simulink model "FTCSimulation_2023a"  (R2023a)
settings: Solver=FixedStepAuto  StartTime=0.0  StopTime=SimTime  FixedStep=0.01  RelTol=1e-3
values from neighbouring files (symbols this model uses):
  g = 9.81    [aero_guid_dat.m]
  Iyy = 182.5/(Kg2slug*m2ft^2)    (= 247.436636441)    [aero_guid_dat.m]
  L = 0.0065    [aero_guid_dat.m]
undefined symbols (not defined in the file or in its folder): A_x, A_y, A_z, AF, apSampleTime, arSampleTime, B_x, B_y, B_z, c_1, c_2, c_3, c_4, C_x, C_y, C_z, CAM, Continuous, D_x, D_y, D_z, Dis, ESO, GOSELM, inertia, Ixx, Izz, K_a1, K_a2, K_a3, K_d, K_d_LQR_phi, K_d_LQR_psi, K_d_LQR_theta, K_d_LQR_x, K_d_LQR_y, K_d_LQR_z, K_p1, K_p2, K_p3, K_q_LQR_phi, K_q_LQR_psi, K_q_LQR_theta, K_q_LQR_x, K_q_LQR_y, K_q_LQR_z, lambda, m, M, Noise, SM, Time
libraries: simulink x6, ctrlSharedLib x3, eeGeneralControl x1
(part 1 of 2)
settings Model: PacingRate=1.400000  Creator=Mahdi  LastModifiedBy=Mahdi
settings OptimizationCC: UseDivisionForNetSlopeComputation=on  GainParamInheritBuiltInType=on  UseFloatMulNetSlope=on  EnhancedBackFolding=on  PassReuseOutputArgsThreshold=0  MaxStackSize=64  OptimizeBlockOrder=speed  DifferentSizesBufferReuse=on  OptimizationCustomize=off
settings DebuggingCC: MultiTaskRateTransMsg=warning  ParameterTunabilityLossMsg=error  UnconnectedInputMsg=warning  UnconnectedOutputMsg=warning  UnconnectedLineMsg=warning
settings ModelReferenceCC: EnableRefExpFcnMdlSchedulingChecks=on
settings SFSimCC: MATLABDynamicMemAlloc=off
settings RTWCC: GenerateReport=on  BuildConfiguration=Faster Runs  LaunchReport=on  DLArmComputeVersion=19.05
settings CodeAppCC: ForceParamTrailComments=on  OperatorAnnotations=on  StateflowObjectComments=on
settings GRTTargetCC: TargetLangStandard=C89/C90 (ANSI)

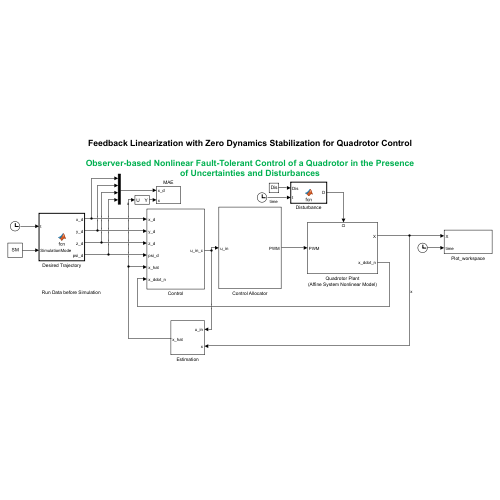
[thumbnail: Simulink's stored preview of the top-level diagram]
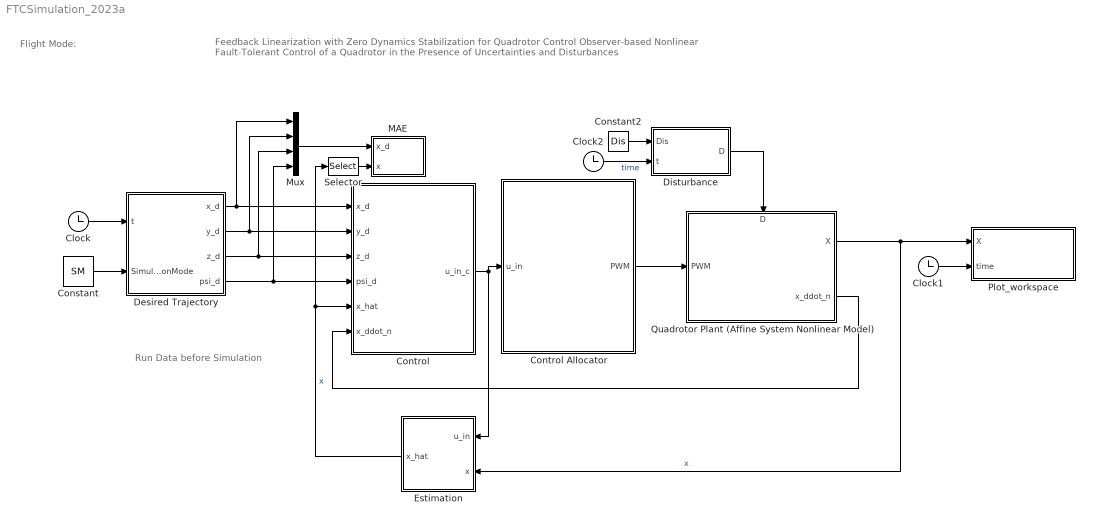
== system FTCSimulation_2023a ==
  note: Run Data before Simulation
  note: Flight Mode:
  note: Feedback Linearization with Zero Dynamics Stabilization for Quadrotor Control
      |
      | Observer-based Nonlinear Fault-Tolerant Control of a Quadrotor in the Presence of Uncertainties and Disturbances
  Clock : Clock
  Clock1 : Clock
  Clock2 : Clock
  Constant : Constant  Value=SM
  Constant2 : Constant  Value=Dis
  Control : Subsystem
  Control Allocator : Subsystem  SystemSampleTime=arSampleTime
  Desired Trajectory : MATLAB Function  TreatAsAtomicUnit=on
  Disturbance : MATLAB Function  TreatAsAtomicUnit=on
  Estimation : Subsystem  VariantControl=true
  MAE : Subsystem
  Mux : Mux
  Plot_workspace : Subsystem
  Quadrotor Plant (Affine System Nonlinear Model) : Subsystem  VariantControl=Choice_1
      settings: PortSchema="{\"entries\":[{\"content\":{\"sides\":[{\"content\":{\"connectorIds\":[\"In1\"]},\"type\":\"ConnectorPlacement.EquallySpacedRectSide\",\"uuid\":\"56cf6a8b-cd11-499a-8a7a-bce78fe94a21\"},{\"content\":{\"connectorIds\":[\"Out1\",\"Out2\"],\"side\":\"RIGHT\"},\"type\":\"ConnectorPlacement.EquallySpacedRectSide\",\"uuid\":\"b8074e7e-b572-4105-951c-798bb82723f6\"},{\"content\":{\"connectorIds\":[\"In2\"],\"side\":\"TOP\"},\"type\":\"ConnectorPlacement.EquallySpacedRectSide\",\"uuid\":\"331d9772-f954-417a-8685-e6b6106d3a97\"}]},\"type\":\"ConnectorPlacement.EquallySpacedConnector\",\"uuid\":\"13cb1b10-b6e3-4763-ba11-23de6fd316ae\"}],\"packageUris\":[\"http://schema.mathworks.com/mf0/Connector/R2020b\"],\"version\":\"1.0\"}"
  Selector : Selector  InputPortWidth=12  IndexOptions=Index vector (dialog)  Indices=[1 2 3 6]  OutputSizes=1
  wires:
  Control/1(u_in_c) -> Estimation/1(u_in), Control Allocator/1(u_in)
  Desired Trajectory/4(psi_d) -> Mux/4, Control/4(psi_d)
  Desired Trajectory/3(z_d) -> Mux/3, Control/3(z_d)
  Desired Trajectory/2(y_d) -> Mux/2, Control/2(y_d)
  Desired Trajectory/1(x_d) -> Mux/1, Control/1(x_d)
  Control Allocator/1(PWM) -> Quadrotor Plant (Affine System Nonlinear Model)/1(PWM)
  Quadrotor Plant (Affine System Nonlinear Model)/1(X) -> Estimation/2(x), Plot_workspace/1(X)  "x"
  Clock/1 -> Desired Trajectory/1(t)
  Constant/1 -> Desired Trajectory/2(SimulationMode)
  Clock1/1 -> Plot_workspace/2(time)
  Clock2/1 -> Disturbance/2(t)  "time"
  Constant2/1 -> Disturbance/1(Dis)
  Disturbance/1(D) -> Quadrotor Plant (Affine System Nonlinear Model)/2(D)
  Quadrotor Plant (Affine System Nonlinear Model)/2(x_ddot_n) -> Control/6(x_ddot_n)
  Estimation/1(x_hat) -> Selector/1, Control/5(x_hat)  "x"
  Mux/1 -> MAE/1(x_d)
  Selector/1 -> MAE/2(x)

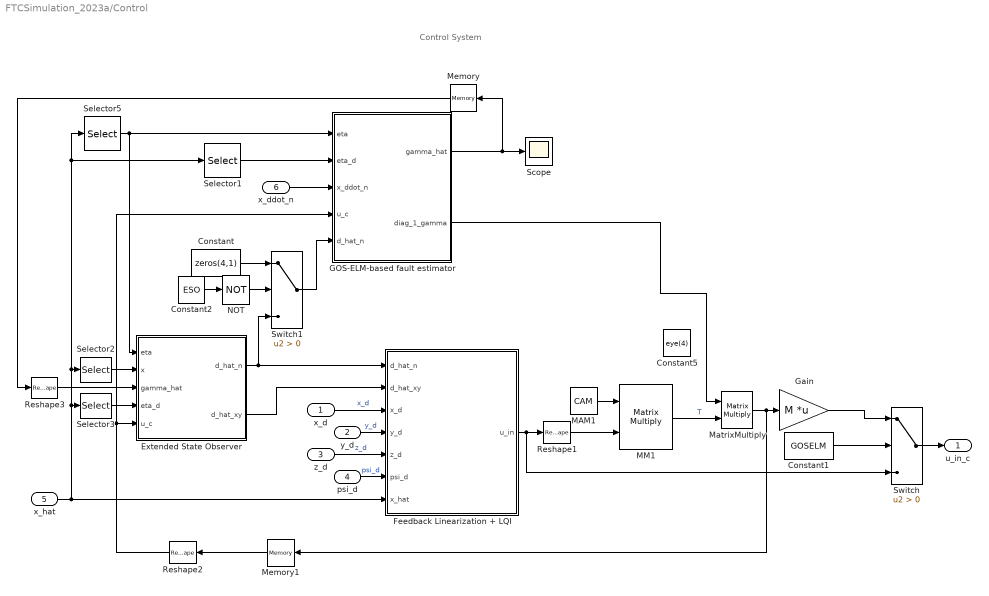
== system FTCSimulation_2023a/Control ==
  note: Control System
  x_d : Inport  OutDataTypeStr=double
  y_d : Inport  Port=2  OutDataTypeStr=double
  z_d : Inport  Port=3  OutDataTypeStr=double
  psi_d : Inport  Port=4
  x_hat : Inport  Port=5
  x_ddot_n : Inport  Port=6
  Constant : Constant  Value=zeros(4,1)
  Constant1 : Constant  Value=GOSELM
  Constant2 : Constant  Value=ESO
  Constant5 : Constant  Value=eye(4)
  Extended State Observer : Subsystem
  Feedback Linearization + LQI : Subsystem
  GOS-ELM-based fault estimator : MATLAB Function  TreatAsAtomicUnit=on
  Gain : Gain  Gain=M  Multiplication=Matrix(K*u)
  MAM1 : Constant  Value=CAM
  MM1 : Product  Multiplication=Matrix(*)  RndMeth=Simplest
  MatrixMultiply : Product  Multiplication=Matrix(*)
  Memory : Memory
  Memory1 : Memory
  NOT : Logic  Operator=NOT  IconShape=distinctive  AllPortsSameDT=off  OutDataTypeStr=boolean
  Reshape1 : Reshape  OutputDimensionality=Column vector (2-D)
  Reshape2 : Reshape  OutputDimensionality=Column vector (2-D)
  Reshape3 : Reshape  OutputDimensionality=Column vector (2-D)
  Scope : Scope
  Selector1 : Selector  InputPortWidth=12  IndexOptions=Index vector (dialog)  Indices=[10 11 12]  OutputSizes=1
  Selector2 : Selector  InputPortWidth=12  IndexOptions=Index vector (dialog)  Indices=[1 2 3]  OutputSizes=1
  Selector3 : Selector  InputPortWidth=12  IndexOptions=Index vector (dialog)  Indices=[10 11 12]  OutputSizes=1
  Selector5 : Selector  InputPortWidth=12  IndexOptions=Index vector (dialog)  Indices=[4 5 6]  OutputSizes=1
  Switch : Switch  Criteria=u2 > Threshold  SaturateOnIntegerOverflow=off  InputSameDT=off
  Switch1 : Switch  Criteria=u2 > Threshold  SaturateOnIntegerOverflow=off  InputSameDT=off
  u_in_c : Outport
  wires:
  x_d/1 -> Feedback Linearization + LQI/3(x_d)  "x_d"
  y_d/1 -> Feedback Linearization + LQI/4(y_d)  "y_d"
  z_d/1 -> Feedback Linearization + LQI/5(z_d)  "z_d"
  psi_d/1 -> Feedback Linearization + LQI/6(psi_d)  "psi_d"
  x_hat/1 -> Selector3/1, Selector1/1, Selector5/1, Selector2/1, Feedback Linearization + LQI/7(x_hat)
  Selector5/1 -> Extended State Observer/1(eta), GOS-ELM-based fault estimator/1(eta)
  Selector1/1 -> GOS-ELM-based fault estimator/2(eta_d)
  x_ddot_n/1 -> GOS-ELM-based fault estimator/3(x_ddot_n)
  Reshape2/1 -> GOS-ELM-based fault estimator/4(u_c), Extended State Observer/5(u_c)
  GOS-ELM-based fault estimator/1(gamma_hat) -> Memory/1, Scope/1
  Reshape1/1 -> MM1/2
  MAM1/1 -> MM1/1
  MM1/1 -> MatrixMultiply/2  "T"
  Gain/1 -> Switch/1
  Constant1/1 -> Switch/2
  Feedback Linearization + LQI/1(u_in) -> Switch/3, Reshape1/1
  Switch/1 -> u_in_c/1
  Constant/1 -> Switch1/1
  Switch1/1 -> GOS-ELM-based fault estimator/5(d_hat_n)
  Constant2/1 -> NOT/1
  NOT/1 -> Switch1/2
  Memory/1 -> Reshape3/1
  MatrixMultiply/1 -> Memory1/1, Gain/1
  Memory1/1 -> Reshape2/1
  Reshape3/1 -> Extended State Observer/3(gamma_hat)
  Selector2/1 -> Extended State Observer/2(x)
  Selector3/1 -> Extended State Observer/4(eta_d)
  Extended State Observer/1(d_hat_n) -> Feedback Linearization + LQI/1(d_hat_n), Switch1/3
  Extended State Observer/2(d_hat_xy) -> Feedback Linearization + LQI/2(d_hat_xy)
  GOS-ELM-based fault estimator/2(diag_1_gamma) -> MatrixMultiply/1

== system FTCSimulation_2023a/Control Allocator ==
  note: Control Allocator (motor mixer)
  u_in : Inport
  MAM : Constant  Value=CAM
  MM : Product  Multiplication=Matrix(*)  RndMeth=Simplest
  Reshape : Reshape  OutputDimensionality=Column vector (2-D)
  RotorThrustToPWM : MATLAB Function  TreatAsAtomicUnit=on
  Saturation : Saturate  UpperLimit=inf  LowerLimit=0
  Saturation1 : Saturate  UpperLimit=100  LowerLimit=0
  Scope{,1..3} (4 alike) : Scope
  PWM : Outport
  wires:
  Reshape/1 -> MM/2
  MM/1 -> Scope3/1, Saturation/1
  MAM/1 -> MM/1
  Saturation/1 -> Scope/1, RotorThrustToPWM/1(T)  "T"
  u_in/1 -> Scope2/1, Reshape/1
  RotorThrustToPWM/1(PWM) -> Scope1/1, Saturation1/1
  Saturation1/1 -> PWM/1

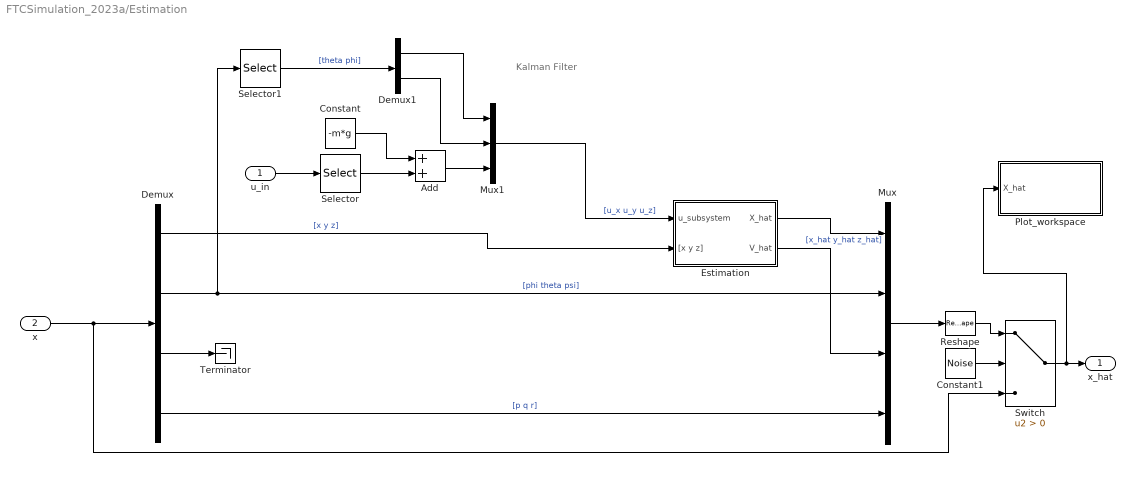
== system FTCSimulation_2023a/Estimation ==
  note: Kalman Filter
  u_in : Inport
  x : Inport  Port=2
  Add : Sum
  Constant : Constant  Value=-m*g
  Constant1 : Constant  Value=Noise
  Demux : Demux
  Demux1 : Demux  Outputs=2
  Estimation : Subsystem
  Mux : Mux
  Mux1 : Mux  Inputs=3
  Plot_workspace : Subsystem
  Reshape : Reshape  OutputDimensionality=Column vector (2-D)
  Selector : Selector  InputPortWidth=4  IndexOptions=Index vector (dialog)  Indices=[1]  OutputSizes=1
  Selector1 : Selector  InputPortWidth=3  IndexOptions=Index vector (dialog)  Indices=[2 1]  OutputSizes=1
  Switch : Switch  Criteria=u2 > Threshold  SaturateOnIntegerOverflow=off  InputSameDT=off
  Terminator : Terminator
  x_hat : Outport
  wires:
  Demux/2 -> Mux/2, Selector1/1  "[phi theta psi]"
  Demux/4 -> Mux/4  "[p q r]"
  Reshape/1 -> Switch/1
  Estimation/1(X_hat) -> Mux/1  "[x_hat y_hat z_hat]"
  Demux/1 -> Estimation/2("[x y z]")  "[x y z]"
  u_in/1 -> Selector/1
  Mux1/1 -> Estimation/1(u_subsystem)  "[u_x u_y u_z]"
  Add/1 -> Mux1/3
  Demux1/1 -> Mux1/1
  Demux1/2 -> Mux1/2
  Selector1/1 -> Demux1/1  "[theta phi]"
  Selector/1 -> Add/2
  Constant/1 -> Add/1
  Mux/1 -> Reshape/1
  Estimation/2(V_hat) -> Mux/3
  Demux/3 -> Terminator/1
  Switch/1 -> Plot_workspace/1(X_hat), x_hat/1
  x/1 -> Switch/3, Demux/1
  Constant1/1 -> Switch/2

== system FTCSimulation_2023a/MAE ==
  x_d : Inport
  x : Inport  Port=2
  Abs : Abs  SaturateOnIntegerOverflow=off
  Clock : Clock
  Display : Display
  Divide : Product  Inputs=*/
  IC : InitialCondition
  Integrator : Integrator
  Scope : Scope
  Subtract : Sum  Inputs=+-
  To Workspace : ToWorkspace  VariableName=MAE  SampleTime=-1
      settings: MaxDataPoints=1
  wires:
  x_d/1 -> Subtract/2
  Subtract/1 -> Abs/1
  Abs/1 -> Integrator/1
  Integrator/1 -> Divide/1
  Divide/1 -> Scope/1, Display/1, To Workspace/1  "MAE"
  Clock/1 -> IC/1
  IC/1 -> Divide/2
  x/1 -> Subtract/1

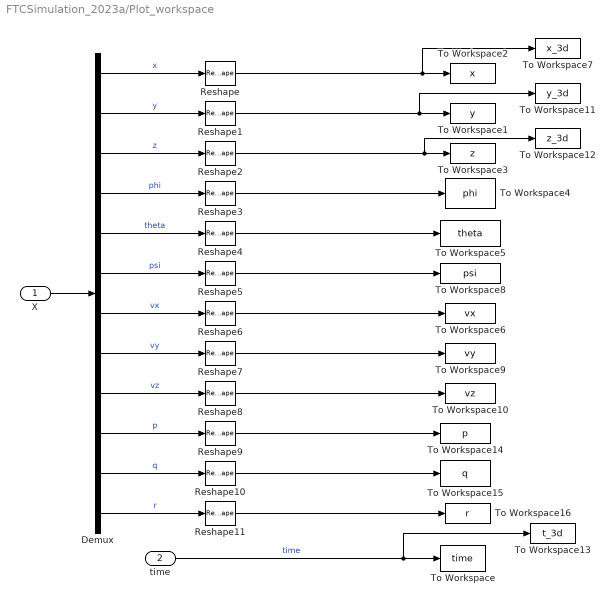
== system FTCSimulation_2023a/Plot_workspace ==
  X : Inport
  time : Inport  Port=2
  Demux : Demux  Outputs=12
  Reshape{,1..11} (12 alike) : Reshape
  To Workspace : ToWorkspace  VariableName=time  SampleTime=-1
      settings: Decimation=5
  To Workspace1 : ToWorkspace  VariableName=y  SampleTime=-1
      settings: Decimation=5
  To Workspace10 : ToWorkspace  VariableName=vz  SampleTime=-1
      settings: Decimation=5
  To Workspace11 : ToWorkspace  VariableName=y_3d  SampleTime=-1
      settings: Decimation=20
  To Workspace12 : ToWorkspace  VariableName=z_3d  SampleTime=-1
      settings: Decimation=20
  To Workspace13 : ToWorkspace  VariableName=t_3d  SampleTime=-1
      settings: Decimation=20
  To Workspace14 : ToWorkspace  VariableName=p  SampleTime=-1
      settings: Decimation=5
  To Workspace15 : ToWorkspace  VariableName=q  SampleTime=-1
      settings: Decimation=5
  To Workspace16 : ToWorkspace  VariableName=r  SampleTime=-1
      settings: Decimation=5
  To Workspace2 : ToWorkspace  VariableName=x  SampleTime=-1
      settings: Decimation=5
  To Workspace3 : ToWorkspace  VariableName=z  SampleTime=-1
      settings: Decimation=5
  To Workspace4 : ToWorkspace  VariableName=phi  SampleTime=-1
      settings: Decimation=5
  To Workspace5 : ToWorkspace  VariableName=theta  SampleTime=-1
      settings: Decimation=5
  To Workspace6 : ToWorkspace  VariableName=vx  SampleTime=-1
      settings: Decimation=5
  To Workspace7 : ToWorkspace  VariableName=x_3d  SampleTime=-1
      settings: Decimation=20
  To Workspace8 : ToWorkspace  VariableName=psi  SampleTime=-1
      settings: Decimation=5
  To Workspace9 : ToWorkspace  VariableName=vy  SampleTime=-1
      settings: Decimation=5
  wires:
  Demux/1 -> Reshape/1  "x"
  Demux/7 -> Reshape6/1  "vx"
  Demux/5 -> Reshape4/1  "theta"
  Demux/10 -> Reshape9/1  "p"
  Demux/9 -> Reshape8/1  "vz"
  Demux/11 -> Reshape10/1  "q"
  Demux/2 -> Reshape1/1  "y"
  Demux/3 -> Reshape2/1  "z"
  Demux/4 -> Reshape3/1  "phi"
  time/1 -> To Workspace13/1, To Workspace/1  "time"
  Demux/8 -> Reshape7/1  "vy"
  Demux/6 -> Reshape5/1  "psi"
  Demux/12 -> Reshape11/1  "r"
  X/1 -> Demux/1
  Reshape/1 -> To Workspace7/1, To Workspace2/1
  Reshape1/1 -> To Workspace11/1, To Workspace1/1
  Reshape2/1 -> To Workspace12/1, To Workspace3/1
  Reshape3/1 -> To Workspace4/1
  Reshape4/1 -> To Workspace5/1
  Reshape5/1 -> To Workspace8/1
  Reshape6/1 -> To Workspace6/1
  Reshape7/1 -> To Workspace9/1
  Reshape8/1 -> To Workspace10/1
  Reshape9/1 -> To Workspace14/1
  Reshape10/1 -> To Workspace15/1
  Reshape11/1 -> To Workspace16/1

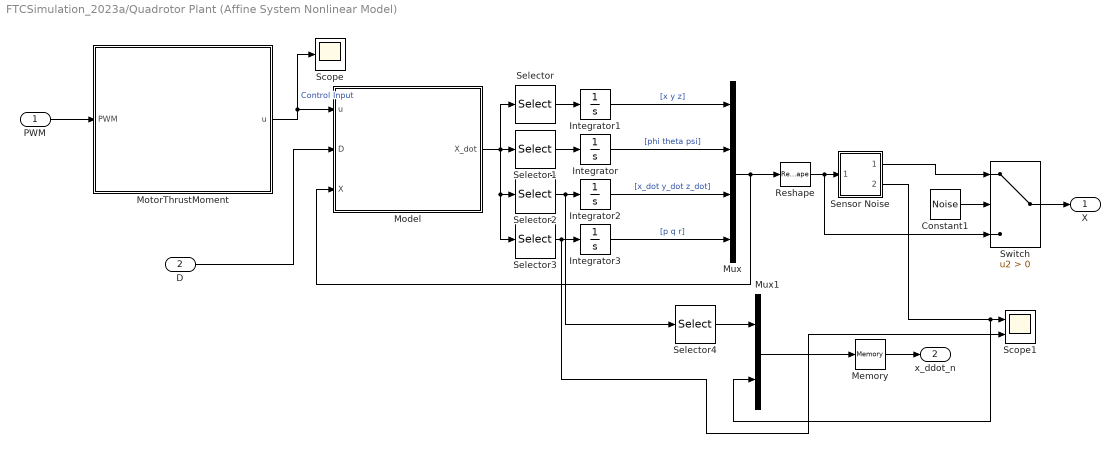
== system FTCSimulation_2023a/Quadrotor Plant (Affine System Nonlinear Model) ==
  PWM : Inport
  D : Inport  Port=2
  Constant1 : Constant  Value=Noise
  Integrator : Integrator  InitialCondition=IC.euler.'  WrapState=on
  Integrator1 : Integrator  InitialCondition=IC.pos.'
  Integrator2 : Integrator  InitialCondition=IC.vb.'
  Integrator3 : Integrator  InitialCondition=IC.angRates.'
  Memory : Memory
  Model : MATLAB Function  TreatAsAtomicUnit=on
  MotorThrustMoment : Subsystem
  Mux : Mux
  Mux1 : Mux  Inputs=2
  Reshape : Reshape  OutputDimensionality=Column vector (2-D)
  Scope : Scope
  Scope1 : Scope  NumInputPorts=2
  Selector : Selector  InputPortWidth=12  IndexOptions=Index vector (dialog)  Indices=[1 2 3]  OutputSizes=1
  Selector1 : Selector  InputPortWidth=12  IndexOptions=Index vector (dialog)  Indices=[4 5 6]  OutputSizes=1
  Selector2 : Selector  InputPortWidth=12  IndexOptions=Index vector (dialog)  Indices=[7 8 9]  OutputSizes=1
  Selector3 : Selector  InputPortWidth=12  IndexOptions=Index vector (dialog)  Indices=[10 11 12]  OutputSizes=1
  Selector4 : Selector  InputPortWidth=3  IndexOptions=Index vector (dialog)  Indices=3  OutputSizes=1
  Sensor Noise : Subsystem
  Switch : Switch  Criteria=u2 > Threshold  SaturateOnIntegerOverflow=off  InputSameDT=off
  X : Outport
  x_ddot_n : Outport  Port=2
  wires:
  PWM/1 -> MotorThrustMoment/1(PWM)
  MotorThrustMoment/1(u) -> Scope/1, Model/1(u)  "Control Input"
  Integrator/1 -> Mux/2  "[phi theta psi]"
  Integrator1/1 -> Mux/1  "[x y z]"
  Selector/1 -> Integrator1/1
  Model/1(X_dot) -> Selector/1, Selector3/1, Selector2/1, Selector1/1
  Selector1/1 -> Integrator/1
  Selector2/1 -> Selector4/1, Integrator2/1
  Selector3/1 -> Scope1/2, Integrator3/1
  Integrator2/1 -> Mux/3  "[x_dot y_dot z_dot]"
  Integrator3/1 -> Mux/4  "[p q r]"
  Mux/1 -> Model/3(X), Reshape/1
  Sensor Noise/1(Out1) -> Switch/1
  Reshape/1 -> Switch/3, Sensor Noise/1(In1)
  Switch/1 -> X/1
  Constant1/1 -> Switch/2
  Selector4/1 -> Mux1/1
  Mux1/1 -> Memory/1
  D/1 -> Model/2(D)
  Memory/1 -> x_ddot_n/1
  Sensor Noise/2(Out2) -> Mux1/2, Scope1/1

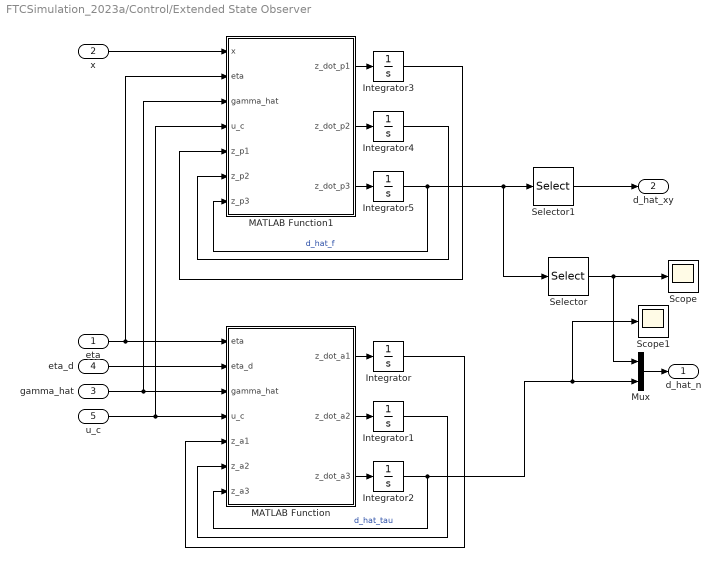
== system FTCSimulation_2023a/Control/Extended State Observer ==
  eta : Inport
  x : Inport  Port=2
  gamma_hat : Inport  Port=3
  eta_d : Inport  Port=4
  u_c : Inport  Port=5
  Integrator{,1..5} (6 alike) : Integrator  InitialCondition=zeros(3,1)
  MATLAB Function : MATLAB Function  TreatAsAtomicUnit=on
  MATLAB Function1 : MATLAB Function  TreatAsAtomicUnit=on
  Mux : Mux  Inputs=2
  Scope : Scope
  Scope1 : Scope
  Selector : Selector  InputPortWidth=3  IndexOptions=Index vector (dialog)  Indices=3  OutputSizes=1
  Selector1 : Selector  InputPortWidth=3  IndexOptions=Index vector (dialog)  Indices=[1 2]  OutputSizes=1
  d_hat_n : Outport
  d_hat_xy : Outport  Port=2
  wires:
  MATLAB Function/1(z_dot_a1) -> Integrator/1
  eta/1 -> MATLAB Function1/2(eta), MATLAB Function/1(eta)
  MATLAB Function/2(z_dot_a2) -> Integrator1/1
  Integrator/1 -> MATLAB Function/5(z_a1)
  Integrator1/1 -> MATLAB Function/6(z_a2)
  MATLAB Function/3(z_dot_a3) -> Integrator2/1
  Integrator2/1 -> MATLAB Function/7(z_a3), Scope1/1, Mux/2  "d_hat_tau"
  Integrator3/1 -> MATLAB Function1/5(z_p1)
  u_c/1 -> MATLAB Function1/4(u_c), MATLAB Function/4(u_c)
  gamma_hat/1 -> MATLAB Function1/3(gamma_hat), MATLAB Function/3(gamma_hat)
  x/1 -> MATLAB Function1/1(x)
  Integrator5/1 -> Selector/1, Selector1/1, MATLAB Function1/7(z_p3)  "d_hat_f"
  Integrator4/1 -> MATLAB Function1/6(z_p2)
  MATLAB Function1/1(z_dot_p1) -> Integrator3/1
  MATLAB Function1/2(z_dot_p2) -> Integrator4/1
  MATLAB Function1/3(z_dot_p3) -> Integrator5/1
  Selector/1 -> Scope/1, Mux/1
  Mux/1 -> d_hat_n/1
  Selector1/1 -> d_hat_xy/1
  eta_d/1 -> MATLAB Function/2(eta_d)

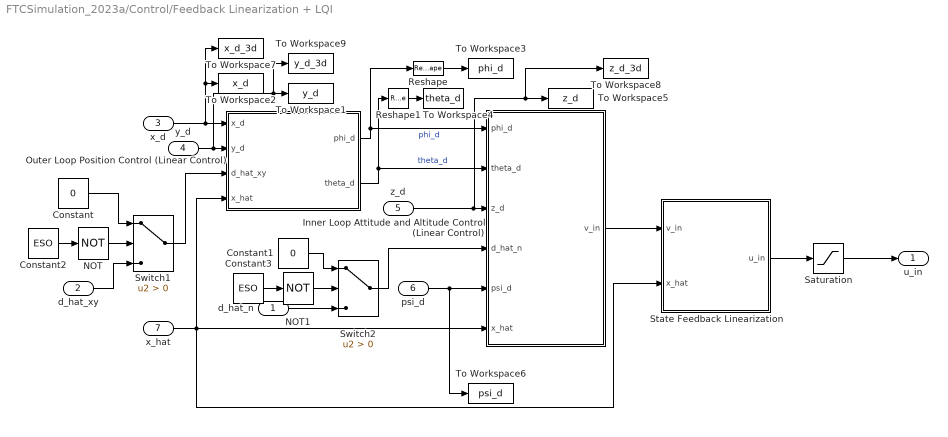
== system FTCSimulation_2023a/Control/Feedback Linearization + LQI ==
  d_hat_n : Inport
  d_hat_xy : Inport  Port=2
  x_d : Inport  Port=3
  y_d : Inport  Port=4
  z_d : Inport  Port=5  OutDataTypeStr=double
  psi_d : Inport  Port=6
  x_hat : Inport  Port=7
  Constant : Constant  Value=0
  Constant1 : Constant  Value=0
  Constant2 : Constant  Value=ESO
  Constant3 : Constant  Value=ESO
  Inner Loop Attitude and Altitude Control (Linear Control) : Subsystem
  NOT : Logic  Operator=NOT  IconShape=distinctive  AllPortsSameDT=off  OutDataTypeStr=boolean
  NOT1 : Logic  Operator=NOT  IconShape=distinctive  AllPortsSameDT=off  OutDataTypeStr=boolean
  Outer Loop Position Control (Linear Control) : Subsystem
  Reshape : Reshape
  Reshape1 : Reshape
  Saturation : Saturate  UpperLimit=[10;0.5;0.5;0.5]  LowerLimit=[0;-0.5;-0.5;-0.5]
  State Feedback Linearization : Subsystem
  Switch1 : Switch  Criteria=u2 > Threshold  SaturateOnIntegerOverflow=off  InputSameDT=off
  Switch2 : Switch  Criteria=u2 > Threshold  SaturateOnIntegerOverflow=off  InputSameDT=off
  To Workspace1 : ToWorkspace  VariableName=y_d  SampleTime=-1
      settings: Decimation=5
  To Workspace2 : ToWorkspace  VariableName=x_d  SampleTime=-1
      settings: Decimation=5
  To Workspace3 : ToWorkspace  VariableName=phi_d  SampleTime=-1
      settings: Decimation=5
  To Workspace4 : ToWorkspace  VariableName=theta_d  SampleTime=-1
      settings: Decimation=5
  To Workspace5 : ToWorkspace  VariableName=z_d  SampleTime=-1
      settings: Decimation=5
  To Workspace6 : ToWorkspace  VariableName=psi_d  SampleTime=-1
      settings: Decimation=5
  To Workspace7 : ToWorkspace  VariableName=x_d_3d  SampleTime=-1
      settings: Decimation=20
  To Workspace8 : ToWorkspace  VariableName=z_d_3d  SampleTime=-1
      settings: Decimation=20
  To Workspace9 : ToWorkspace  VariableName=y_d_3d  SampleTime=-1
      settings: Decimation=20
  u_in : Outport
  wires:
  x_d/1 -> To Workspace7/1, To Workspace2/1, Outer Loop Position Control (Linear Control)/1(x_d)
  y_d/1 -> To Workspace9/1, To Workspace1/1, Outer Loop Position Control (Linear Control)/2(y_d)
  Inner Loop Attitude and Altitude Control (Linear Control)/1(v_in) -> State Feedback Linearization/1(v_in)
  Outer Loop Position Control (Linear Control)/1(phi_d) -> Inner Loop Attitude and Altitude Control (Linear Control)/1(phi_d), Reshape/1  "phi_d"
  Outer Loop Position Control (Linear Control)/2(theta_d) -> Inner Loop Attitude and Altitude Control (Linear Control)/2(theta_d), Reshape1/1  "theta_d"
  x_hat/1 -> Outer Loop Position Control (Linear Control)/4(x_hat), State Feedback Linearization/2(x_hat), Inner Loop Attitude and Altitude Control (Linear Control)/6(x_hat)
  z_d/1 -> To Workspace8/1, To Workspace5/1, Inner Loop Attitude and Altitude Control (Linear Control)/3(z_d)
  Reshape/1 -> To Workspace3/1
  State Feedback Linearization/1(u_in) -> Saturation/1
  psi_d/1 -> To Workspace6/1, Inner Loop Attitude and Altitude Control (Linear Control)/5(psi_d)
  Reshape1/1 -> To Workspace4/1
  Saturation/1 -> u_in/1
  Constant2/1 -> NOT/1
  NOT/1 -> Switch1/2
  d_hat_xy/1 -> Switch1/3
  Switch1/1 -> Outer Loop Position Control (Linear Control)/3(d_hat_xy)
  Constant/1 -> Switch1/1
  Constant1/1 -> Switch2/1
  NOT1/1 -> Switch2/2
  Constant3/1 -> NOT1/1
  d_hat_n/1 -> Switch2/3
  Switch2/1 -> Inner Loop Attitude and Altitude Control (Linear Control)/4(d_hat_n)

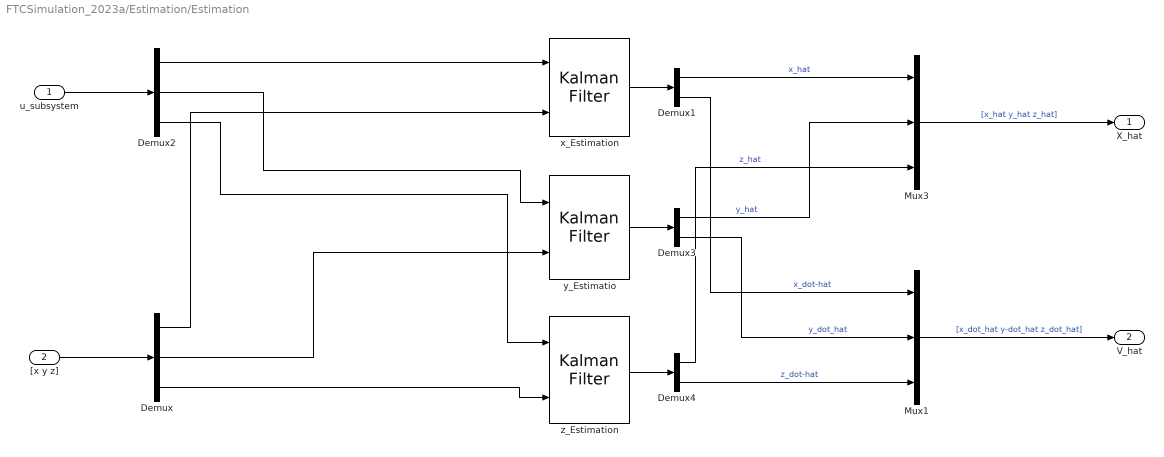
== system FTCSimulation_2023a/Estimation/Estimation ==
  u_subsystem : Inport
  "[x y z]" : Inport  Port=2
  Demux : Demux  Outputs=3
  Demux1 : Demux  Outputs=2
  Demux2 : Demux  Outputs=3
  Demux3 : Demux  Outputs=2
  Demux4 : Demux  Outputs=2
  Mux1 : Mux  Inputs=3
  Mux3 : Mux  Inputs=3
  x_Estimation : ctrlSharedLib/Kalman Filter  TimeDomain=Continuous-Time  UseCurrentEstimator=on  ModelSource=Individual A, B, C, D matrices  ModelSourceVariable=ss(0.95,1,1,0,1)  A=A_x  B=B_x  C=C_x  D=D_x  NumberOfStates=1  NumberOfInputs=1  NumberOfOutputs=1  InitialEstimateSource=Dialog  X0=0  P0=10  UseK=off  UseGH=off  NumberOfProcessNoiseInputs=1  G=1  TimeInvariantG=on  H=0  TimeInvariantH=on  Q=diag([10^(-11) , 1.25*10^(-10)])  TimeInvariantQ=on  R=0.1  TimeInvariantR=on  N=0  TimeInvariantN=on  AddInputPort=on  AddEnablePort=off  OutputEstimatedY=off  OutputP=off  Ts=0.01
  y_Estimatio : ctrlSharedLib/Kalman Filter  TimeDomain=Continuous-Time  UseCurrentEstimator=on  ModelSource=Individual A, B, C, D matrices  ModelSourceVariable=ss(0.95,1,1,0,1)  A=A_y  B=B_y  C=C_y  D=D_y  NumberOfStates=1  NumberOfInputs=1  NumberOfOutputs=1  InitialEstimateSource=Dialog  X0=0  P0=10  UseK=off  UseGH=off  NumberOfProcessNoiseInputs=1  G=1  TimeInvariantG=on  H=0  TimeInvariantH=on  Q=diag([10^(-11),25*10^(-11)])  TimeInvariantQ=on  R=[1.25*10^(-7)]  TimeInvariantR=on  N=0  TimeInvariantN=on  AddInputPort=on  AddEnablePort=off  OutputEstimatedY=off  OutputP=off  Ts=0.01
  z_Estimation : ctrlSharedLib/Kalman Filter  TimeDomain=Continuous-Time  UseCurrentEstimator=on  ModelSource=Individual A, B, C, D matrices  ModelSourceVariable=ss(0.95,1,1,0,1)  A=A_z  B=B_z  C=C_z  D=D_z  NumberOfStates=1  NumberOfInputs=1  NumberOfOutputs=1  InitialEstimateSource=Dialog  X0=0  P0=10  UseK=off  UseGH=off  NumberOfProcessNoiseInputs=1  G=1  TimeInvariantG=on  H=0  TimeInvariantH=on  Q=diag([25*10^(-9),4*10^(-9)])  TimeInvariantQ=on  R=[1.25*10^(-8)]  TimeInvariantR=on  N=0  TimeInvariantN=on  AddInputPort=on  AddEnablePort=off  OutputEstimatedY=off  OutputP=off  Ts=0.01
  X_hat : Outport
  V_hat : Outport  Port=2
  wires:
  "[x y z]"/1 -> Demux/1
  Demux/1 -> x_Estimation/2
  Demux/2 -> y_Estimatio/2
  Demux/3 -> z_Estimation/2
  u_subsystem/1 -> Demux2/1
  Demux2/1 -> x_Estimation/1
  Demux2/2 -> y_Estimatio/1
  Demux2/3 -> z_Estimation/1
  Mux3/1 -> X_hat/1  "[x_hat y_hat z_hat]"
  x_Estimation/1 -> Demux1/1
  Demux1/1 -> Mux3/1  "x_hat"
  Demux3/1 -> Mux3/2  "y_hat"
  z_Estimation/1 -> Demux4/1
  Demux4/1 -> Mux3/3  "z_hat"
  y_Estimatio/1 -> Demux3/1
  Demux4/2 -> Mux1/3  "z_dot-hat"
  Demux3/2 -> Mux1/2  "y_dot_hat"
  Demux1/2 -> Mux1/1  "x_dot-hat"
  Mux1/1 -> V_hat/1  "[x_dot_hat y-dot_hat z_dot_hat]"

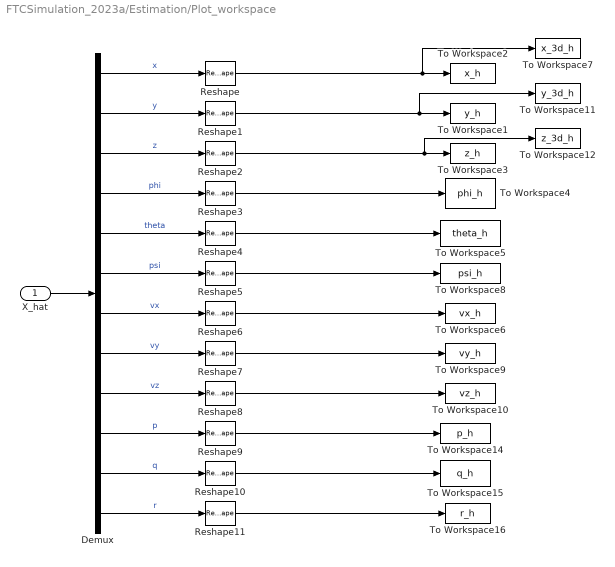
== system FTCSimulation_2023a/Estimation/Plot_workspace ==
  X_hat : Inport
  Demux : Demux  Outputs=12
  Reshape{,1..11} (12 alike) : Reshape
  To Workspace1 : ToWorkspace  VariableName=y_h  SampleTime=-1
      settings: Decimation=5
  To Workspace10 : ToWorkspace  VariableName=vz_h  SampleTime=-1
      settings: Decimation=5
  To Workspace11 : ToWorkspace  VariableName=y_3d_h  SampleTime=-1
      settings: Decimation=20
  To Workspace12 : ToWorkspace  VariableName=z_3d_h  SampleTime=-1
      settings: Decimation=20
  To Workspace14 : ToWorkspace  VariableName=p_h  SampleTime=-1
      settings: Decimation=5
  To Workspace15 : ToWorkspace  VariableName=q_h  SampleTime=-1
      settings: Decimation=5
  To Workspace16 : ToWorkspace  VariableName=r_h  SampleTime=-1
      settings: Decimation=5
  To Workspace2 : ToWorkspace  VariableName=x_h  SampleTime=-1
      settings: Decimation=5
  To Workspace3 : ToWorkspace  VariableName=z_h  SampleTime=-1
      settings: Decimation=5
  To Workspace4 : ToWorkspace  VariableName=phi_h  SampleTime=-1
      settings: Decimation=5
  To Workspace5 : ToWorkspace  VariableName=theta_h  SampleTime=-1
      settings: Decimation=5
  To Workspace6 : ToWorkspace  VariableName=vx_h  SampleTime=-1
      settings: Decimation=5
  To Workspace7 : ToWorkspace  VariableName=x_3d_h  SampleTime=-1
      settings: Decimation=20
  To Workspace8 : ToWorkspace  VariableName=psi_h  SampleTime=-1
      settings: Decimation=5
  To Workspace9 : ToWorkspace  VariableName=vy_h  SampleTime=-1
      settings: Decimation=5
  wires:
  Demux/1 -> Reshape/1  "x"
  Demux/7 -> Reshape6/1  "vx"
  Demux/5 -> Reshape4/1  "theta"
  Demux/10 -> Reshape9/1  "p"
  Demux/9 -> Reshape8/1  "vz"
  Demux/11 -> Reshape10/1  "q"
  Demux/2 -> Reshape1/1  "y"
  Demux/3 -> Reshape2/1  "z"
  Demux/4 -> Reshape3/1  "phi"
  Demux/8 -> Reshape7/1  "vy"
  Demux/6 -> Reshape5/1  "psi"
  Demux/12 -> Reshape11/1  "r"
  X_hat/1 -> Demux/1
  Reshape/1 -> To Workspace7/1, To Workspace2/1
  Reshape1/1 -> To Workspace11/1, To Workspace1/1
  Reshape2/1 -> To Workspace12/1, To Workspace3/1
  Reshape3/1 -> To Workspace4/1
  Reshape4/1 -> To Workspace5/1
  Reshape5/1 -> To Workspace8/1
  Reshape6/1 -> To Workspace6/1
  Reshape7/1 -> To Workspace9/1
  Reshape8/1 -> To Workspace10/1
  Reshape9/1 -> To Workspace14/1
  Reshape10/1 -> To Workspace15/1
  Reshape11/1 -> To Workspace16/1

== system FTCSimulation_2023a/Quadrotor Plant (Affine System Nonlinear Model)/MotorThrustMoment ==
  note: Motors Configuration
  PWM : Inport
  Actuator Fault : MATLAB Function  TreatAsAtomicUnit=on
  Clock : Clock
  Constant : Constant  Value=[70 70 70 70]
  Constant1 : Constant  Value=[6;0;0;0]
  Constant3 : Constant  Value=AF
  Gain : Gain  Gain=M  Multiplication=Matrix(K*u)
  Manual Switch : ManualSwitch
  Manual Switch1 : ManualSwitch
  MotorThrust : Subsystem
  Mux : Mux
  Reshape1 : Reshape  OutputDimensionality=Column vector (2-D)
  u : Outport
  wires:
  PWM/1 -> Manual Switch/1
  MotorThrust/1(T1) -> Mux/1
  MotorThrust/2(T2) -> Mux/2
  MotorThrust/3(T3) -> Mux/3
  MotorThrust/4(T4) -> Mux/4
  Reshape1/1 -> Gain/1
  Gain/1 -> Manual Switch1/1
  Manual Switch/1 -> MotorThrust/1(PWM)
  Constant/1 -> Manual Switch/2
  Manual Switch1/1 -> u/1
  Constant1/1 -> Manual Switch1/2
  Constant3/1 -> Actuator Fault/1(AF)
  Clock/1 -> Actuator Fault/3(t)
  Mux/1 -> Actuator Fault/2(u_c)
  Actuator Fault/1(u) -> Reshape1/1

== system FTCSimulation_2023a/Quadrotor Plant (Affine System Nonlinear Model)/Sensor Noise ==
  In1 : Inport
  Demux : Demux
  Filtered Derivative (Discrete or Continuous) : eeGeneralControl/Filtered Derivative (Discrete or Continuous)  K=1  T=0.1  B=inf  A=-inf  minRatio=10  init_option=Inherited from block input  x0=0  Ts=-1
      settings: LibrarySourceBlock=|
      | ee_sl_lib/General Control/Filtered Derivative
      | (Discrete or Continuous)
  Mux : Mux
  Reshape : Reshape  OutputDimensionality=Column vector (2-D)
  Subsystem : Subsystem
  Subsystem3 : Subsystem
  Out1 : Outport
  Out2 : Outport  Port=2
  wires:
  In1/1 -> Demux/1
  Demux/1 -> Subsystem/1(In1)  "[x y z["
  Demux/2 -> Mux/2  "[phi theta psi]"
  Demux/3 -> Mux/3  "[x_dot y_dot z_dot]"
  Demux/4 -> Subsystem3/1(In1)  "[p q r]"
  Subsystem/1(Out1) -> Mux/1
  Subsystem3/1(Out1) -> Filtered Derivative (Discrete or Continuous)/1, Mux/4
  Mux/1 -> Reshape/1
  Reshape/1 -> Out1/1
  Filtered Derivative (Discrete or Continuous)/1 -> Out2/1

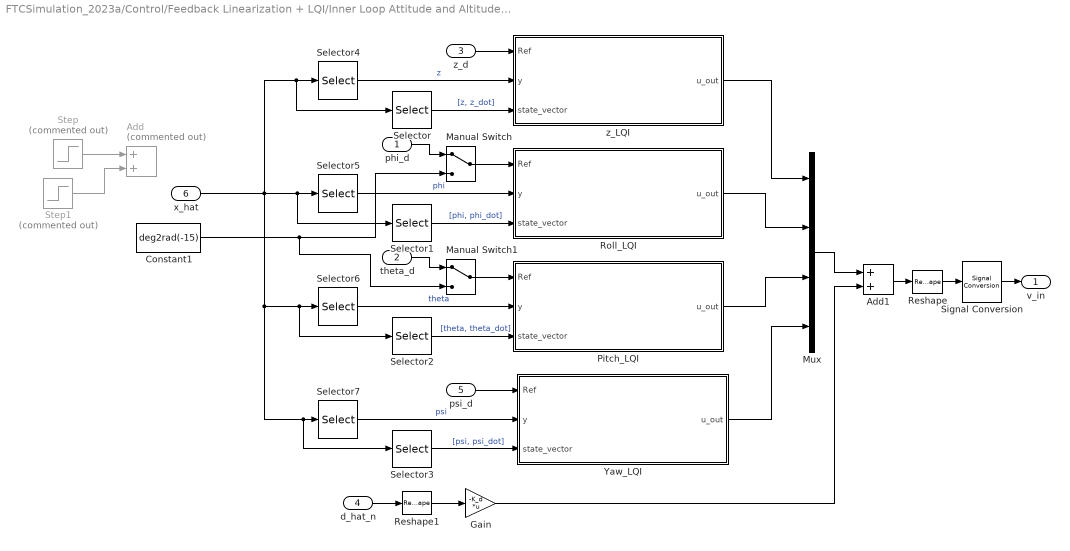
== system FTCSimulation_2023a/Control/Feedback Linearization + LQI/Inner Loop Attitude and Altitude Control (Linear Control) ==
  phi_d : Inport
  theta_d : Inport  Port=2
  z_d : Inport  Port=3
  d_hat_n : Inport  Port=4
  psi_d : Inport  Port=5
  x_hat : Inport  Port=6
  Add : Sum  Commented=on
  Add1 : Sum
  Constant1 : Constant  Value=deg2rad(-15)
  Gain : Gain  Gain=-K_d  Multiplication=Matrix(K*u)
  Manual Switch : ManualSwitch
  Manual Switch1 : ManualSwitch
  Mux : Mux
  Pitch_LQI : Subsystem  mask{K_d=K_d_LQR_theta, InitialCondition=0, K_i=-K_q_LQR_theta}
      mask prompts: K_d "State Feedback Gain (K):"; InitialCondition "Initial Condition for Integrator:"; K_i "Integral Gain (K_i):"
      mask TypeOptions K_d: k_d/Gain
      mask TypeOptions InitialCondition: Integrator4/InitialCondition
      mask TypeOptions K_i: k_i/Gain
      mask Display: disp('Linear-Quadratic-Integral control\n (LQI)');
  Reshape : Reshape  OutputDimensionality=Column vector (2-D)
  Reshape1 : Reshape  OutputDimensionality=Column vector (2-D)
  Roll_LQI : Subsystem  mask{K_d=K_d_LQR_phi, InitialCondition=0, K_i=-K_q_LQR_phi}
      mask prompts: K_d "State Feedback Gain (K):"; InitialCondition "Initial Condition for Integrator:"; K_i "Integral Gain (K_i):"
      mask TypeOptions K_d: k_d/Gain
      mask TypeOptions InitialCondition: Integrator4/InitialCondition
      mask TypeOptions K_i: k_i/Gain
      mask Display: disp('Linear-Quadratic-Integral control\n (LQI)');
  Selector : Selector  InputPortWidth=12  IndexOptions=Index vector (dialog)  Indices=[3 9]  OutputSizes=1
  Selector1 : Selector  InputPortWidth=12  IndexOptions=Index vector (dialog)  Indices=[4 10]  OutputSizes=1
  Selector2 : Selector  InputPortWidth=12  IndexOptions=Index vector (dialog)  Indices=[5 11]  OutputSizes=1
  Selector3 : Selector  InputPortWidth=12  IndexOptions=Index vector (dialog)  Indices=[6 12]  OutputSizes=1
  Selector4 : Selector  InputPortWidth=12  IndexOptions=Index vector (dialog)  Indices=3  OutputSizes=1
  Selector5 : Selector  InputPortWidth=12  IndexOptions=Index vector (dialog)  Indices=4  OutputSizes=1
  Selector6 : Selector  InputPortWidth=12  IndexOptions=Index vector (dialog)  Indices=5  OutputSizes=1
  Selector7 : Selector  InputPortWidth=12  IndexOptions=Index vector (dialog)  Indices=6  OutputSizes=1
  Signal Conversion : SignalConversion  OverrideOpt=off
  Step : Step  Commented=on  Time=25  After=0.2  SampleTime=0
  Step1 : Step  Commented=on  Time=40  After=-0.1  SampleTime=0
  Yaw_LQI : Subsystem  mask{K_d=K_d_LQR_psi, InitialCondition=0, K_i=-K_q_LQR_psi}
      mask prompts: K_d "State Feedback Gain (K):"; InitialCondition "Initial Condition for Integrator:"; K_i "Integral Gain (K_i):"
      mask TypeOptions K_d: k_d/Gain
      mask TypeOptions InitialCondition: Integrator4/InitialCondition
      mask TypeOptions K_i: k_i/Gain
      mask Display: disp('Linear-Quadratic-Integral control\n (LQI)');
  z_LQI : Subsystem  mask{K_d=K_d_LQR_z, InitialCondition=0, K_i=-K_q_LQR_z}
      mask prompts: K_d "State Feedback Gain (K):"; InitialCondition "Initial Condition for Integrator:"; K_i "Integral Gain (K_i):"
      mask TypeOptions K_d: k_d/Gain
      mask TypeOptions InitialCondition: Integrator4/InitialCondition
      mask TypeOptions K_i: k_i/Gain
      mask Display: disp('Linear-Quadratic-Integral control\n (LQI)');
  v_in : Outport
  wires:
  z_d/1 -> z_LQI/1(Ref)
  psi_d/1 -> Yaw_LQI/1(Ref)
  Selector/1 -> z_LQI/3(state_vector)  "[z, z_dot]"
  x_hat/1 -> Selector/1, Selector4/1, Selector7/1, Selector3/1, Selector6/1, Selector2/1, Selector5/1, Selector1/1
  Selector1/1 -> Roll_LQI/3(state_vector)  "[phi, phi_dot]"
  Selector2/1 -> Pitch_LQI/3(state_vector)  "[theta, theta_dot]"
  Selector3/1 -> Yaw_LQI/3(state_vector)  "[psi, psi_dot]"
  Selector4/1 -> z_LQI/2(y)  "z"
  Selector5/1 -> Roll_LQI/2(y)  "phi"
  Selector6/1 -> Pitch_LQI/2(y)  "theta"
  Selector7/1 -> Yaw_LQI/2(y)  "psi"
  z_LQI/1(u_out) -> Mux/1
  Roll_LQI/1(u_out) -> Mux/2
  Pitch_LQI/1(u_out) -> Mux/3
  Yaw_LQI/1(u_out) -> Mux/4
  Mux/1 -> Add1/1
  Reshape/1 -> Signal Conversion/1
  Signal Conversion/1 -> v_in/1
  Manual Switch/1 -> Roll_LQI/1(Ref)
  phi_d/1 -> Manual Switch/1
  Manual Switch1/1 -> Pitch_LQI/1(Ref)
  theta_d/1 -> Manual Switch1/1
  Step/1 -> Add/1
  Step1/1 -> Add/2
  Constant1/1 -> Manual Switch1/2, Manual Switch/2
  d_hat_n/1 -> Reshape1/1
  Gain/1 -> Add1/2
  Add1/1 -> Reshape/1
  Reshape1/1 -> Gain/1

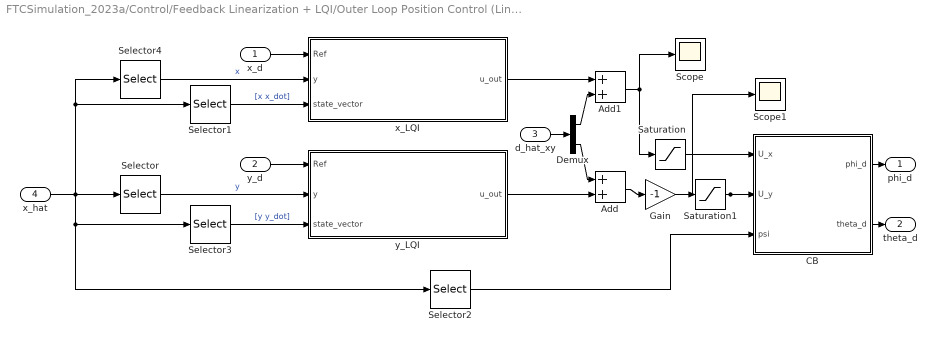
== system FTCSimulation_2023a/Control/Feedback Linearization + LQI/Outer Loop Position Control (Linear Control) ==
  x_d : Inport
  y_d : Inport  Port=2
  d_hat_xy : Inport  Port=3
  x_hat : Inport  Port=4
  Add : Sum
  Add1 : Sum
  CB : Subsystem  SystemSampleTime=apSampleTime
  Demux : Demux  Outputs=2
  Gain : Gain  Gain=-1
  Saturation : Saturate  UpperLimit=0.2  LowerLimit=-0.2
  Saturation1 : Saturate  UpperLimit=0.2  LowerLimit=-0.2
  Scope : Scope
  Scope1 : Scope
  Selector : Selector  InputPortWidth=12  IndexOptions=Index vector (dialog)  Indices=2  OutputSizes=1
  Selector1 : Selector  InputPortWidth=12  IndexOptions=Index vector (dialog)  Indices=[1 7]  OutputSizes=1
  Selector2 : Selector  InputPortWidth=12  IndexOptions=Index vector (dialog)  Indices=6  OutputSizes=1
  Selector3 : Selector  InputPortWidth=12  IndexOptions=Index vector (dialog)  Indices=[2 8]  OutputSizes=1
  Selector4 : Selector  InputPortWidth=12  IndexOptions=Index vector (dialog)  Indices=1  OutputSizes=1
  x_LQI : Subsystem  mask{K_d=K_d_LQR_x, InitialCondition=0, K_i=-K_q_LQR_x}
      mask prompts: K_d "State Feedback Gain (K):"; InitialCondition "Initial Condition for Integrator:"; K_i "Integral Gain (K_i):"
      mask TypeOptions K_d: k_d/Gain
      mask TypeOptions InitialCondition: Integrator4/InitialCondition
      mask TypeOptions K_i: k_i/Gain
      mask Display: disp('Linear-Quadratic-Integral control\n (LQI)');
  y_LQI : Subsystem  mask{K_d=K_d_LQR_y, InitialCondition=0, K_i=-K_q_LQR_y}
      mask prompts: K_d "State Feedback Gain (K):"; InitialCondition "Initial Condition for Integrator:"; K_i "Integral Gain (K_i):"
      mask TypeOptions K_d: k_d/Gain
      mask TypeOptions InitialCondition: Integrator4/InitialCondition
      mask TypeOptions K_i: k_i/Gain
      mask Display: disp('Linear-Quadratic-Integral control\n (LQI)');
  phi_d : Outport
  theta_d : Outport  Port=2
  wires:
  CB/1(phi_d) -> phi_d/1
  CB/2(theta_d) -> theta_d/1
  x_hat/1 -> Selector2/1, Selector3/1, Selector1/1, Selector4/1, Selector/1
  Selector2/1 -> CB/3(psi)
  x_d/1 -> x_LQI/1(Ref)
  y_d/1 -> y_LQI/1(Ref)
  Selector/1 -> y_LQI/2(y)  "y"
  Selector4/1 -> x_LQI/2(y)  "x"
  Selector1/1 -> x_LQI/3(state_vector)  "[x x_dot]"
  Selector3/1 -> y_LQI/3(state_vector)  "[y y_dot]"
  Add1/1 -> Saturation/1, Scope/1
  Add/1 -> Gain/1
  Saturation/1 -> CB/1(U_x)
  Saturation1/1 -> Scope1/1, CB/2(U_y)
  Gain/1 -> Saturation1/1
  y_LQI/1(u_out) -> Add/2
  x_LQI/1(u_out) -> Add1/1
  d_hat_xy/1 -> Demux/1
  Demux/1 -> Add1/2
  Demux/2 -> Add/1

== system FTCSimulation_2023a/Control/Feedback Linearization + LQI/State Feedback Linearization ==
  v_in : Inport
  x_hat : Inport  Port=2
  Constant : Constant  Value=Ixx
  Constant1 : Constant  Value=Iyy
  Constant2 : Constant  Value=Izz
  Constant3 : Constant  Value=g
  Constant4 : Constant  Value=m
  MATLAB Function : MATLAB Function  TreatAsAtomicUnit=on
  u_in : Outport
  wires:
  v_in/1 -> MATLAB Function/1(v_in)
  MATLAB Function/1(u_in) -> u_in/1
  x_hat/1 -> MATLAB Function/2(x_hat)
  Constant/1 -> MATLAB Function/3(Ix)
  Constant1/1 -> MATLAB Function/4(Iy)
  Constant2/1 -> MATLAB Function/5(Iz)
  Constant3/1 -> MATLAB Function/6(g)
  Constant4/1 -> MATLAB Function/7(m)

== system FTCSimulation_2023a/Quadrotor Plant (Affine System Nonlinear Model)/MotorThrustMoment/MotorThrust ==
  PWM : Inport
  Demux : Demux
  PWM_To_Thrust1 : Subsystem  mask{a=1.14e-4, b=1.018e-2, Value=6.5833e-2}
      mask prompts: Value "c:"
      mask TypeOptions a: a/Gain
      mask TypeOptions b: b/Gain
      mask TypeOptions Value: c/Value
      mask DialogControl DescTextVar Prompt: Motor Thrust Quadratic Relation with PWM
      mask DialogControl Control2 Prompt: T = a*PWM^2+b*PWM+c
  PWM_To_Thrust2 : Subsystem  mask{a=1.1544e-4, b=7.7509e-3, Value=9.5961e-2}
      mask prompts: Value "c:"
      mask TypeOptions a: a/Gain
      mask TypeOptions b: b/Gain
      mask TypeOptions Value: c/Value
      mask DialogControl DescTextVar Prompt: Motor Thrust Quadratic Relation with PWM
      mask DialogControl Control2 Prompt: T = a*PWM^2+b*PWM+c
  PWM_To_Thrust3 : Subsystem  mask{a=1.2605e-4, b=9.2952e-3, Value=7.214e-2}
      mask prompts: Value "c:"
      mask TypeOptions a: a/Gain
      mask TypeOptions b: b/Gain
      mask TypeOptions Value: c/Value
      mask DialogControl DescTextVar Prompt: Motor Thrust Quadratic Relation with PWM
      mask DialogControl Control2 Prompt: T = a*PWM^2+b*PWM+c
  PWM_To_Thrust4 : Subsystem  mask{a=1.3045e-4, b=7.5567e-3, Value=8.2877e-2}
      mask prompts: Value "c:"
      mask TypeOptions a: a/Gain
      mask TypeOptions b: b/Gain
      mask TypeOptions Value: c/Value
      mask DialogControl DescTextVar Prompt: Motor Thrust Quadratic Relation with PWM
      mask DialogControl Control2 Prompt: T = a*PWM^2+b*PWM+c
  T1 : Outport
  T2 : Outport  Port=2
  T3 : Outport  Port=3
  T4 : Outport  Port=4
  wires:
  PWM/1 -> Demux/1
  Demux/1 -> PWM_To_Thrust1/1(PWM1)
  Demux/2 -> PWM_To_Thrust2/1(PWM2)
  Demux/3 -> PWM_To_Thrust3/1(PWM3)
  Demux/4 -> PWM_To_Thrust4/1(PWM4)
  PWM_To_Thrust1/1(T1) -> T1/1
  PWM_To_Thrust2/1(T2) -> T2/1
  PWM_To_Thrust3/1(T3) -> T3/1
  PWM_To_Thrust4/1(T4) -> T4/1

== system FTCSimulation_2023a/Quadrotor Plant (Affine System Nonlinear Model)/Sensor Noise/Subsystem ==
  In1 : Inport
  Add : Sum
  Add1 : Sum
  Add2 : Sum
  Band-Limited White Noise : simulink/Sources/Band-Limited White Noise  Cov=[1.25*10^(-10)]  Ts=0.01  seed=[23341]
  Band-Limited White Noise1 : simulink/Sources/Band-Limited White Noise  Cov=[1.51*10^(-10)]  Ts=0.01  seed=[23342]
  Band-Limited White Noise2 : simulink/Sources/Band-Limited White Noise  Cov=[1.18*10^(-8)]  Ts=0.01  seed=[23343]
  Demux : Demux  Outputs=3
  Mux : Mux  Inputs=3
  Out1 : Outport
  wires:
  In1/1 -> Demux/1
  Demux/1 -> Add/2
  Band-Limited White Noise/1 -> Add/1
  Add/1 -> Mux/1
  Add1/1 -> Mux/2
  Demux/2 -> Add1/2
  Band-Limited White Noise1/1 -> Add1/1
  Add2/1 -> Mux/3
  Band-Limited White Noise2/1 -> Add2/1
  Demux/3 -> Add2/2
  Mux/1 -> Out1/1

== system FTCSimulation_2023a/Quadrotor Plant (Affine System Nonlinear Model)/Sensor Noise/Subsystem3 ==
  In1 : Inport
  Add : Sum
  Add1 : Sum
  Add2 : Sum
  Band-Limited White Noise : simulink/Sources/Band-Limited White Noise  Cov=[4*10^(-6)]  Ts=0.01  seed=[23341]
  Band-Limited White Noise1 : simulink/Sources/Band-Limited White Noise  Cov=[3*10^(-6)]  Ts=0.01  seed=[23342]
  Band-Limited White Noise2 : simulink/Sources/Band-Limited White Noise  Cov=[2*10^(-6)]  Ts=0.01  seed=[23343]
  Demux : Demux  Outputs=3
  Mux : Mux  Inputs=3
  Out1 : Outport
  wires:
  Add2/1 -> Mux/3
  Add1/1 -> Mux/2
  Demux/1 -> Add/2
  Add/1 -> Mux/1
  Mux/1 -> Out1/1
  Band-Limited White Noise/1 -> Add/1
  In1/1 -> Demux/1
  Band-Limited White Noise2/1 -> Add2/1
  Demux/2 -> Add1/2
  Demux/3 -> Add2/2
  Band-Limited White Noise1/1 -> Add1/1

== system FTCSimulation_2023a/Control/Feedback Linearization + LQI/Inner Loop Attitude and Altitude Control (Linear Control)/Pitch_LQI ==
  Ref : Inport
  y : Inport  Port=2
  state_vector : Inport  Port=3
  Integrator4 : Integrator  InitialCondition=InitialCondition
  Reshape1 : Reshape  OutputDimensionality=Column vector (2-D)
  Reshape2 : Reshape  OutputDimensionality=Column vector (2-D)
  Reshape3 : Reshape  OutputDimensionality=Column vector (2-D)
  Sum10 : Sum  Inputs=|+-
  Sum12 : Sum  Inputs=|+-
  k_d : Gain  Gain=K_d  Multiplication=Matrix(K*u)
  k_i : Gain  Gain=K_i  Multiplication=Matrix(K*u)
  u_out : Outport
  wires:
  k_i/1 -> Sum10/1  "-Kixi"
  Integrator4/1 -> k_i/1  "xi"
  Reshape2/1 -> k_d/1
  Sum12/1 -> Integrator4/1  "e = xi_dot"
  state_vector/1 -> Reshape2/1
  k_d/1 -> Sum10/2  "K_dx"
  Sum10/1 -> u_out/1
  Reshape1/1 -> Sum12/1
  Ref/1 -> Reshape1/1
  Reshape3/1 -> Sum12/2
  y/1 -> Reshape3/1

== system FTCSimulation_2023a/Control/Feedback Linearization + LQI/Inner Loop Attitude and Altitude Control (Linear Control)/Roll_LQI ==
  Ref : Inport
  y : Inport  Port=2
  state_vector : Inport  Port=3
  Integrator4 : Integrator  InitialCondition=InitialCondition
  Reshape1 : Reshape  OutputDimensionality=Column vector (2-D)
  Reshape2 : Reshape  OutputDimensionality=Column vector (2-D)
  Reshape3 : Reshape  OutputDimensionality=Column vector (2-D)
  Sum10 : Sum  Inputs=|+-
  Sum12 : Sum  Inputs=|+-
  k_d : Gain  Gain=K_d  Multiplication=Matrix(K*u)
  k_i : Gain  Gain=K_i  Multiplication=Matrix(K*u)
  u_out : Outport
  wires:
  y/1 -> Reshape3/1
  Reshape3/1 -> Sum12/2
  Ref/1 -> Reshape1/1
  Reshape1/1 -> Sum12/1
  Sum10/1 -> u_out/1
  k_d/1 -> Sum10/2  "K_dx"
  state_vector/1 -> Reshape2/1
  Sum12/1 -> Integrator4/1  "e = xi_dot"
  Reshape2/1 -> k_d/1
  Integrator4/1 -> k_i/1  "xi"
  k_i/1 -> Sum10/1  "-Kixi"

== system FTCSimulation_2023a/Control/Feedback Linearization + LQI/Inner Loop Attitude and Altitude Control (Linear Control)/Yaw_LQI ==
  Ref : Inport
  y : Inport  Port=2
  state_vector : Inport  Port=3
  Integrator4 : Integrator  InitialCondition=InitialCondition
  Reshape1 : Reshape  OutputDimensionality=Column vector (2-D)
  Reshape2 : Reshape  OutputDimensionality=Column vector (2-D)
  Reshape3 : Reshape  OutputDimensionality=Column vector (2-D)
  Sum10 : Sum  Inputs=|+-
  Sum12 : Sum  Inputs=|+-
  k_d : Gain  Gain=K_d  Multiplication=Matrix(K*u)
  k_i : Gain  Gain=K_i  Multiplication=Matrix(K*u)
  u_out : Outport
  wires:
  y/1 -> Reshape3/1
  Reshape3/1 -> Sum12/2
  Ref/1 -> Reshape1/1
  Reshape1/1 -> Sum12/1
  Sum10/1 -> u_out/1
  k_d/1 -> Sum10/2  "K_dx"
  state_vector/1 -> Reshape2/1
  Sum12/1 -> Integrator4/1  "e = xi_dot"
  Reshape2/1 -> k_d/1
  Integrator4/1 -> k_i/1  "xi"
  k_i/1 -> Sum10/1  "-Kixi"

== system FTCSimulation_2023a/Control/Feedback Linearization + LQI/Inner Loop Attitude and Altitude Control (Linear Control)/z_LQI ==
  Ref : Inport
  y : Inport  Port=2
  state_vector : Inport  Port=3
  Integrator4 : Integrator  InitialCondition=InitialCondition
  Reshape1 : Reshape  OutputDimensionality=Column vector (2-D)
  Reshape2 : Reshape  OutputDimensionality=Column vector (2-D)
  Reshape3 : Reshape  OutputDimensionality=Column vector (2-D)
  Sum10 : Sum  Inputs=|+-
  Sum12 : Sum  Inputs=|+-
  k_d : Gain  Gain=K_d  Multiplication=Matrix(K*u)
  k_i : Gain  Gain=K_i  Multiplication=Matrix(K*u)
  u_out : Outport
  wires:
  k_i/1 -> Sum10/1  "-Kixi"
  Integrator4/1 -> k_i/1  "xi"
  Reshape2/1 -> k_d/1
  Sum12/1 -> Integrator4/1  "e = xi_dot"
  state_vector/1 -> Reshape2/1
  k_d/1 -> Sum10/2  "K_dx"
  Sum10/1 -> u_out/1
  Reshape1/1 -> Sum12/1
  Ref/1 -> Reshape1/1
  Reshape3/1 -> Sum12/2
  y/1 -> Reshape3/1

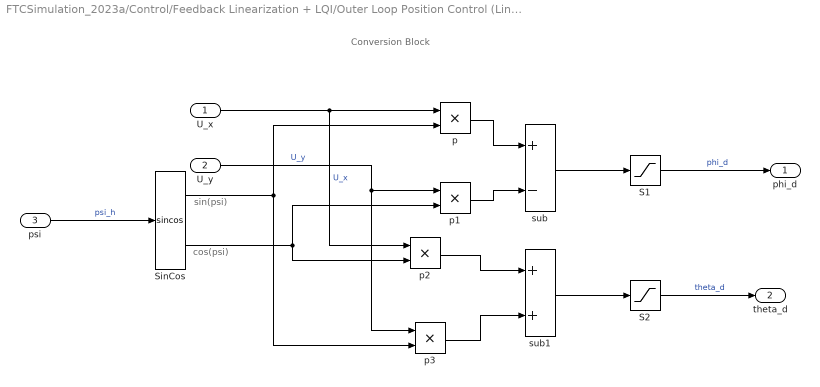
== system FTCSimulation_2023a/Control/Feedback Linearization + LQI/Outer Loop Position Control (Linear Control)/CB ==
  note: cos(psi)
  note: sin(psi)
  note: Conversion Block
  U_x : Inport
  U_y : Inport  Port=2
  psi : Inport  Port=3
  S1 : Saturate  UpperLimit=deg2rad(20)  LowerLimit=-deg2rad(20)  RndMeth=Simplest
  S2 : Saturate  UpperLimit=deg2rad(20)  LowerLimit=-deg2rad(20)  RndMeth=Simplest
  SinCos : Trigonometry  Operator=sincos
  p{,1..3} (4 alike) : Product  RndMeth=Simplest
  sub : Sum  Inputs=+-  RndMeth=Simplest
  sub1 : Sum  RndMeth=Simplest
  phi_d : Outport
  theta_d : Outport  Port=2
  wires:
  U_x/1 -> p2/1, p/1  "U_x"
  p1/1 -> sub/2
  SinCos/2 -> p2/2, p1/2
  p/1 -> sub/1
  S1/1 -> phi_d/1  "phi_d"
  S2/1 -> theta_d/1  "theta_d"
  p3/1 -> sub1/2
  p2/1 -> sub1/1
  U_y/1 -> p1/1, p3/1  "U_y"
  SinCos/1 -> p3/2, p/2
  psi/1 -> SinCos/1  "psi_h"
  sub/1 -> S1/1
  sub1/1 -> S2/1

== system FTCSimulation_2023a/Control/Feedback Linearization + LQI/Outer Loop Position Control (Linear Control)/x_LQI ==
  Ref : Inport
  y : Inport  Port=2
  state_vector : Inport  Port=3
  Integrator4 : Integrator  InitialCondition=InitialCondition
  Reshape1 : Reshape  OutputDimensionality=Column vector (2-D)
  Reshape2 : Reshape  OutputDimensionality=Column vector (2-D)
  Reshape3 : Reshape  OutputDimensionality=Column vector (2-D)
  Sum10 : Sum  Inputs=|+-
  Sum12 : Sum  Inputs=|+-
  k_d : Gain  Gain=K_d  Multiplication=Matrix(K*u)
  k_i : Gain  Gain=K_i  Multiplication=Matrix(K*u)
  u_out : Outport
  wires:
  y/1 -> Reshape3/1
  Reshape3/1 -> Sum12/2
  Ref/1 -> Reshape1/1
  Reshape1/1 -> Sum12/1
  Sum10/1 -> u_out/1
  k_d/1 -> Sum10/2  "K_dx"
  state_vector/1 -> Reshape2/1
  Sum12/1 -> Integrator4/1  "e = xi_dot"
  Reshape2/1 -> k_d/1
  Integrator4/1 -> k_i/1  "xi"
  k_i/1 -> Sum10/1  "-Kixi"

== system FTCSimulation_2023a/Control/Feedback Linearization + LQI/Outer Loop Position Control (Linear Control)/y_LQI ==
  Ref : Inport
  y : Inport  Port=2
  state_vector : Inport  Port=3
  Integrator4 : Integrator  InitialCondition=InitialCondition
  Reshape1 : Reshape  OutputDimensionality=Column vector (2-D)
  Reshape2 : Reshape  OutputDimensionality=Column vector (2-D)
  Reshape3 : Reshape  OutputDimensionality=Column vector (2-D)
  Sum10 : Sum  Inputs=|+-
  Sum12 : Sum  Inputs=|+-
  k_d : Gain  Gain=K_d  Multiplication=Matrix(K*u)
  k_i : Gain  Gain=K_i  Multiplication=Matrix(K*u)
  u_out : Outport
  wires:
  k_i/1 -> Sum10/1  "-Kixi"
  Integrator4/1 -> k_i/1  "xi"
  Reshape2/1 -> k_d/1
  Sum12/1 -> Integrator4/1  "e = xi_dot"
  state_vector/1 -> Reshape2/1
  k_d/1 -> Sum10/2  "K_dx"
  Sum10/1 -> u_out/1
  Reshape1/1 -> Sum12/1
  Ref/1 -> Reshape1/1
  Reshape3/1 -> Sum12/2
  y/1 -> Reshape3/1

== system FTCSimulation_2023a/Quadrotor Plant (Affine System Nonlinear Model)/MotorThrustMoment/MotorThrust/PWM_To_Thrust1 ==
  PWM1 : Inport
  Add : Sum  Inputs=+++
  Math Function : Math  Operator=square
  a : Gain  Gain=a
  b : Gain  Gain=b
  c : Constant  Value=Value
  T1 : Outport
  wires:
  PWM1/1 -> b/1, Math Function/1
  Math Function/1 -> a/1
  a/1 -> Add/1
  b/1 -> Add/2
  c/1 -> Add/3
  Add/1 -> T1/1

== system FTCSimulation_2023a/Quadrotor Plant (Affine System Nonlinear Model)/MotorThrustMoment/MotorThrust/PWM_To_Thrust2 ==
  PWM2 : Inport
  Add : Sum  Inputs=+++
  Math Function : Math  Operator=square
  a : Gain  Gain=a
  b : Gain  Gain=b
  c : Constant  Value=Value
  T2 : Outport
  wires:
  Add/1 -> T2/1
  c/1 -> Add/3
  b/1 -> Add/2
  a/1 -> Add/1
  Math Function/1 -> a/1
  PWM2/1 -> Math Function/1, b/1

== system FTCSimulation_2023a/Quadrotor Plant (Affine System Nonlinear Model)/MotorThrustMoment/MotorThrust/PWM_To_Thrust3 ==
  PWM3 : Inport
  Add : Sum  Inputs=+++
  Math Function : Math  Operator=square
  a : Gain  Gain=a
  b : Gain  Gain=b
  c : Constant  Value=Value
  T3 : Outport
  wires:
  PWM3/1 -> b/1, Math Function/1
  Math Function/1 -> a/1
  a/1 -> Add/1
  b/1 -> Add/2
  c/1 -> Add/3
  Add/1 -> T3/1

== system FTCSimulation_2023a/Quadrotor Plant (Affine System Nonlinear Model)/MotorThrustMoment/MotorThrust/PWM_To_Thrust4 ==
  PWM4 : Inport
  Add : Sum  Inputs=+++
  Math Function : Math  Operator=square
  a : Gain  Gain=a
  b : Gain  Gain=b
  c : Constant  Value=Value
  T4 : Outport
  wires:
  Add/1 -> T4/1
  c/1 -> Add/3
  b/1 -> Add/2
  a/1 -> Add/1
  Math Function/1 -> a/1
  PWM4/1 -> Math Function/1, b/1

== matlab function FTCSimulation_2023a/Control/Extended State Observer/MATLAB Function ==
  data: eta input size=[3 1]; eta_d input; gamma_hat input size=[4 1]; z_dot_a1 output; u_c input size=[4 1]; z_a1 input; z_a2 input; z_a3 input; z_dot_a2 output; z_dot_a3 output; K_a1 parameter; K_a2 parameter; K_a3 parameter; inertia parameter; L parameter; c_1 parameter; c_2 parameter; c_3 parameter; c_4 parameter
function [z_dot_a1,z_dot_a2, z_dot_a3] = fcn(eta,eta_d,gamma_hat,u_c,z_a1,z_a2,z_a3, K_a1, K_a2, K_a3, inertia, L, c_1, c_2, c_3, c_4)

g_nl = [L/inertia(1,1) -L/inertia(1,1) -L/inertia(1,1) L/inertia(1,1);
    -L/inertia(2,2) -L/inertia(2,2) L/inertia(2,2) L/inertia(2,2);
    c_1/inertia(3,3) -c_2/inertia(3,3) c_3/inertia(3,3) -c_4/inertia(3,3)];

e_a1 = eta-z_a1;
z_dot_a1 = z_a2+K_a1*e_a1;
z_dot_a2 = [(inertia(2,2)-inertia(3,3))*eta_d(2)*eta_d(3)/(inertia(1,1));
    (inertia(3,3)-inertia(1,1))*eta_d(1)*eta_d(3)/(inertia(2,2));
    (inertia(1,1)-inertia(2,2))*eta_d(1)*eta_d(2)/(inertia(3,3))] +...
    inv(inertia)*(g_nl*diag(u_c)*gamma_hat)+inv(inertia)*z_a3+K_a2*e_a1;
z_dot_a3 = K_a3*e_a1;

== matlab function FTCSimulation_2023a/Control/Extended State Observer/MATLAB Function1 ==
  data: x input; eta input; gamma_hat input; z_dot_p1 output; u_c input; z_p1 input; z_p2 input; z_p3 input; z_dot_p2 output; z_dot_p3 output; K_p1 parameter; K_p2 parameter; K_p3 parameter; g parameter; m parameter
function [z_dot_p1,z_dot_p2, z_dot_p3] = fcn(x,eta,gamma_hat,u_c,z_p1,z_p2,z_p3, K_p1, K_p2, K_p3, g, m)
Re3 = [cos(eta(1))*sin(eta(2))*cos(eta(3))+sin(eta(1))*sin(eta(3));
       cos(eta(1))*sin(eta(2))*sin(eta(3))-sin(eta(1))*cos(eta(3));
       cos(eta(1))*cos(eta(2))];
T = u_c.'*gamma_hat;
e_p1 = x-z_p1;
z_dot_p1 = z_p2+K_p1*e_p1;
z_dot_p2 = -g*[0;0;1] +(Re3*T+z_p3)/m+ K_p2*e_p1;
z_dot_p3 = K_p3*e_p1;
